simulink model "qConj"  (R2018a)
settings: Solver=VariableStepAuto  StartTime=0.0  StopTime=10.0  RelTol=1e-3
settings Model: Creator=henry  LastModifiedBy=henry

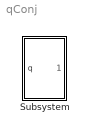
== system qConj ==
  Subsystem : Subsystem  mask(Quaternion Conjugate){}
      mask help: This block takes the conjugate of the input quaternion

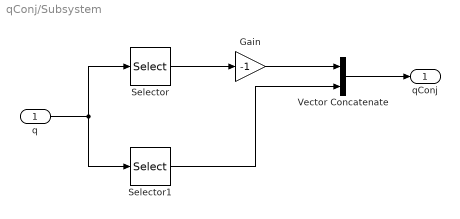
== system qConj/Subsystem ==
  q : Inport
  Gain : Gain  Gain=-1
  Selector : Selector  InputPortWidth=4  IndexOptions=Index vector (dialog)  Indices=[1:3]  OutputSizes=1
  Selector1 : Selector  InputPortWidth=4  IndexOptions=Index vector (dialog)  Indices=4  OutputSizes=1
  Vector Concatenate : Concatenate
  qConj : Outport
  wires:
  Vector Concatenate/1 -> qConj/1
  Gain/1 -> Vector Concatenate/1
  Selector1/1 -> Vector Concatenate/2
  q/1 -> Selector1/1, Selector/1
  Selector/1 -> Gain/1
